simulink model "bridge"  (R2022a)
settings: Solver=VariableStepAuto  StartTime=0.0  StopTime=10.0  RelTol=1e-3
settings Model: Creator=kasturkoul  LastModifiedBy=kasturkoul

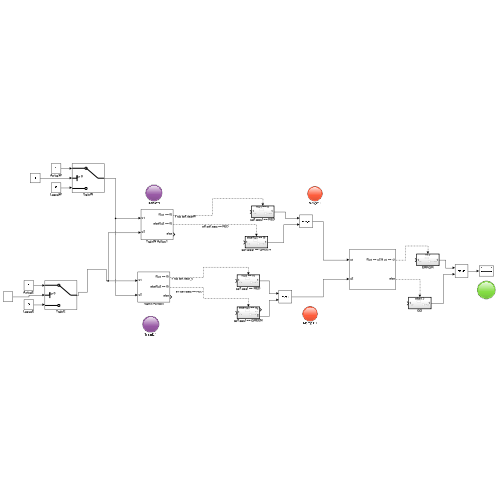
[thumbnail: Simulink's stored preview of the top-level diagram]
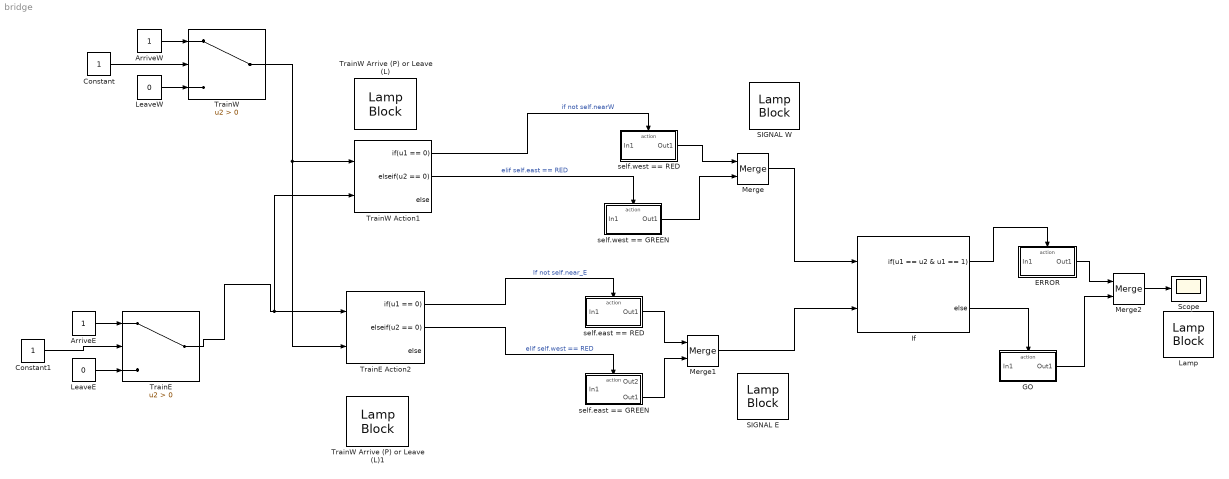
== system bridge ==
  ArriveE : Constant
  ArriveW : Constant
  Constant : Constant
  Constant1 : Constant
  ERROR : Subsystem  TreatAsAtomicUnit=on
  GO : Subsystem  TreatAsAtomicUnit=on
  If : If  NumInputs=2  IfExpression=u1 == u2 & u1 == 1
  Lamp : LampBlock  LabelPosition=Hide
  LeaveE : Constant  Value=0
  LeaveW : Constant  Value=0
  Merge : Merge
  Merge1 : Merge
  Merge2 : Merge
  SIGNAL E : LampBlock  LabelPosition=Bottom
  SIGNAL W : LampBlock  LabelPosition=Bottom
  Scope : Scope
  TrainE : Switch  Criteria=u2 > Threshold  SaturateOnIntegerOverflow=off  InputSameDT=off
  TrainE Action2 : If  NumInputs=2  IfExpression=u1 == 0  ElseIfExpressions=u2 == 0
  TrainW : Switch  Criteria=u2 > Threshold  SaturateOnIntegerOverflow=off  InputSameDT=off
  TrainW Action1 : If  NumInputs=2  IfExpression=u1 == 0  ElseIfExpressions=u2 == 0
  TrainW Arrive (P) or Leave (L) : LampBlock  LabelPosition=Bottom
  TrainW Arrive (P) or Leave (L)1 : LampBlock  LabelPosition=Bottom
  self.east == GREEN : Subsystem  TreatAsAtomicUnit=on
  self.east == RED : Subsystem  TreatAsAtomicUnit=on
  self.west == GREEN : Subsystem  TreatAsAtomicUnit=on
  self.west == RED : Subsystem  TreatAsAtomicUnit=on
  wires:
  ArriveW/1 -> TrainW/1
  LeaveW/1 -> TrainW/3
  TrainW/1 -> TrainE Action2/2, TrainW Action1/1
  Constant/1 -> TrainW/2
  TrainE/1 -> TrainE Action2/1, TrainW Action1/2
  Constant1/1 -> TrainE/2
  ArriveE/1 -> TrainE/1
  LeaveE/1 -> TrainE/3
  TrainW Action1/1 -> self.west == RED/Action  "if not self.nearW"
  TrainW Action1/2 -> self.west == GREEN/Action  "elif self.east == RED"
  TrainE Action2/1 -> self.east == RED/Action  "If not self.near_E"
  TrainE Action2/2 -> self.east == GREEN/Action  "elif self.west == RED"
  self.west == RED/1(Out1) -> Merge/1
  self.west == GREEN/1(Out1) -> Merge/2
  self.east == RED/1(Out1) -> Merge1/1
  self.east == GREEN/2(Out1) -> Merge1/2
  Merge1/1 -> If/2
  Merge/1 -> If/1
  If/1 -> ERROR/Action
  If/2 -> GO/Action
  ERROR/1(Out1) -> Merge2/1
  GO/1(Out1) -> Merge2/2
  Merge2/1 -> Scope/1

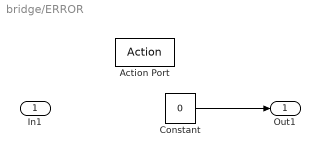
== system bridge/ERROR ==
  In1 : Inport
  Action Port : ActionPort  ActionPortLabel=if(u1 == u2 & u1 == 1)
  Constant : Constant  Value=0
  Out1 : Outport
  wires:
  Constant/1 -> Out1/1

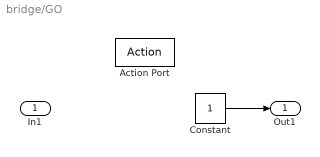
== system bridge/GO ==
  In1 : Inport
  Action Port : ActionPort  ActionPortLabel=else
  Constant : Constant
  Out1 : Outport
  wires:
  Constant/1 -> Out1/1

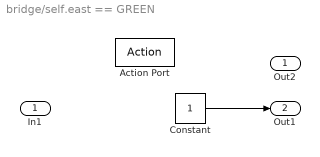
== system bridge/self.east == GREEN ==
  In1 : Inport
  Action Port : ActionPort  ActionPortLabel=elseif(u2 == 0)
  Constant : Constant
  Out2 : Outport
  Out1 : Outport  Port=2
  wires:
  Constant/1 -> Out1/1

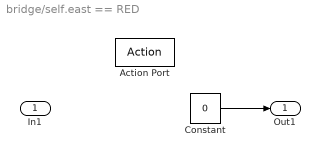
== system bridge/self.east == RED ==
  In1 : Inport
  Action Port : ActionPort  ActionPortLabel=if(u1 == 0)
  Constant : Constant  Value=0
  Out1 : Outport
  wires:
  Constant/1 -> Out1/1

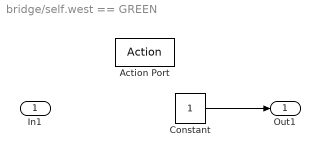
== system bridge/self.west == GREEN ==
  In1 : Inport
  Action Port : ActionPort  ActionPortLabel=elseif(u2 == 0)
  Constant : Constant
  Out1 : Outport
  wires:
  Constant/1 -> Out1/1

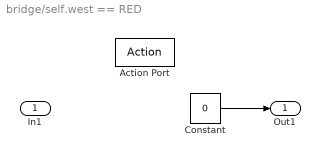
== system bridge/self.west == RED ==
  In1 : Inport
  Action Port : ActionPort  ActionPortLabel=if(u1 == 0)
  Constant : Constant  Value=0
  Out1 : Outport
  wires:
  Constant/1 -> Out1/1
